simulink model "Simulink_Model"  (R2021a)
settings: Solver=VariableStepAuto  StartTime=0.0  StopTime=inf  FixedStep=1  RelTol=1e-3
model workspace (MAT data in the model file):
  M = 1200
  R = 1
libraries: pid_lib x1, simulink x1
settings Model: EnablePacing=on  Creator=matteopenlington  LastModifiedBy=matteopenlington
settings DebuggingCC: UnderSpecifiedDimensionMsg=warning

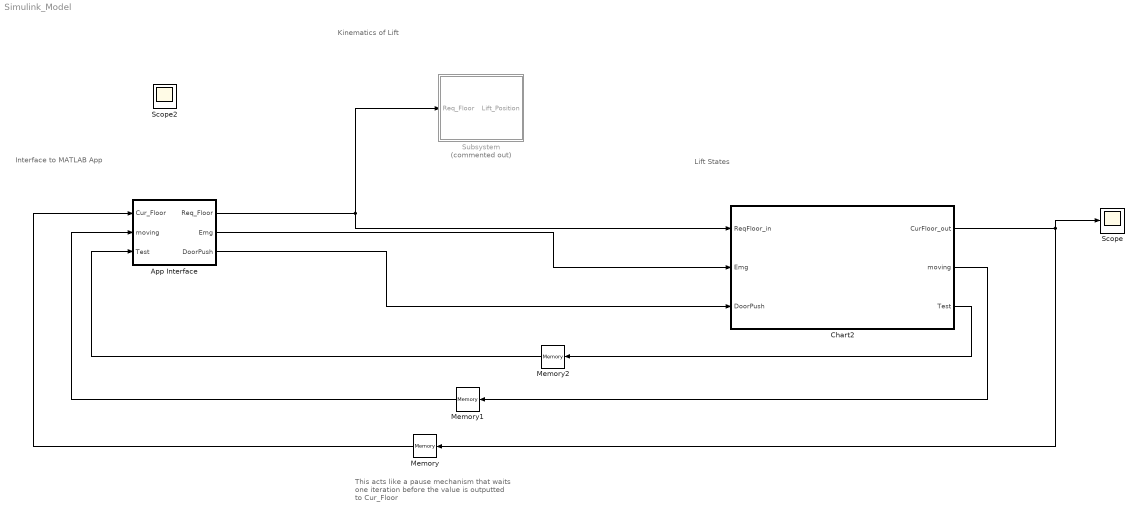
== system Simulink_Model ==
  note: Lift States
  note: Kinematics of Lift
  note: This acts like a pause mechanism that waits one iteration before the value is outputted to Cur_Floor
  note: Interface to MATLAB App
  App Interface : Stateflow chart  TreatAsAtomicUnit=on
  Chart2 : Stateflow chart  TreatAsAtomicUnit=on
  Memory : Memory
  Memory1 : Memory
  Memory2 : Memory
  Scope : Scope
  Subsystem : Subsystem  Commented=on
  Scope2 : Scope
  wires:
  Memory/1 -> App Interface/1(Cur_Floor)
  Chart2/1(CurFloor_out) -> Scope/1, Memory/1
  App Interface/2(Emg) -> Chart2/2(Emg)
  Chart2/2(moving) -> Memory1/1
  Memory1/1 -> App Interface/2(moving)
  App Interface/3(DoorPush) -> Chart2/3(DoorPush)
  Chart2/3(Test) -> Memory2/1
  Memory2/1 -> App Interface/3(Test)
  App Interface/1(Req_Floor) -> Subsystem/1(Req_Floor), Chart2/1(ReqFloor_in)

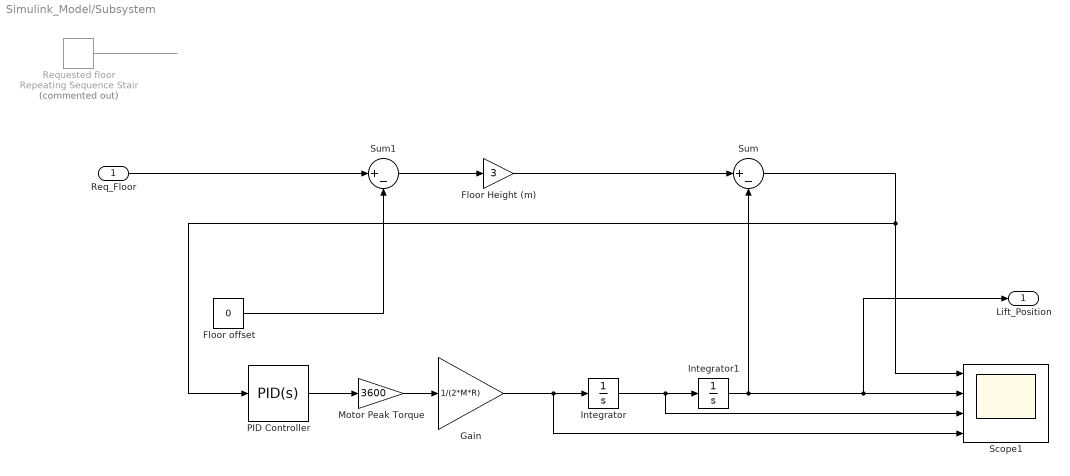
== system Simulink_Model/Subsystem ==
  Req_Floor : Inport
  Floor Height (m) : Gain  Gain=3
  Floor offset : Constant  Value=0
  Gain : Gain  Gain=1/(2*M*R)
  Integrator : Integrator
  Integrator1 : Integrator
  Motor Peak Torque : Gain  Gain=3600
  PID Controller : pid_lib/PID Controller  Controller=PID  Form=Parallel  TimeDomain=Continuous-time  UseExternalTs=off  SampleTime=-1  IntegratorMethod=Forward Euler  FilterMethod=Forward Euler  ControllerParametersSource=internal  P=1  I=0  D=2  UseFilter=on  N=5.45  TunerSelectOption=Transfer Function Based (PID Tuner App)  InitialConditionSource=internal  InitialConditionForIntegrator=0  InitialConditionForFilter=0  DifferentiatorICPrevScaledInput=0  ExternalReset=none  TrackingMode=off  Kt=1  LimitOutput=on  SatLimitsSource=internal  UpperSaturationLimit=1  LowerSaturationLimit=-1  LinearizeAsGain=on  AntiWindupMode=none  Kb=1  POutMin=[]  POutMax=[]  IOutMin=[]  IOutMax=[]  DOutMin=[]  DOutMax=[]  NOutMin=[]  NOutMax=[]  SumOutMin=[]  SumOutMax=[]  SaturationOutMin=[]  SaturationOutMax=[]  PParamMin=[]  PParamMax=[]  IParamMin=[]  IParamMax=[]  DParamMin=[]  DParamMax=[]  NParamMin=[]  NParamMax=[]  KbParamMin=[]  KbParamMax=[]  KtParamMin=[]  KtParamMax=[]  KbOutMin=[]  KbOutMax=[]  KtOutMin=[]  KtOutMax=[]  IntegratorOutMin=[]  IntegratorOutMax=[]  FilterOutMin=[]  FilterOutMax=[]  SumI1OutMin=[]  SumI1OutMax=[]  SumI2OutMin=[]  SumI2OutMax=[]  SumI3OutMin=[]  SumI3OutMax=[]  SumI4OutMin=[]  SumI4OutMax=[]  SumDOutMin=[]  SumDOutMax=[]  DifferentiatorOutMin=[]  DifferentiatorOutMax=[]  FilterDiffOutCoefMin=[]  FilterDiffOutCoefMax=[]  ReciprocalOutMin=[]  ReciprocalOutMax=[]  SumDenOutMin=[]  SumDenOutMax=[]  SumNumOutMin=[]  SumNumOutMax=[]  DivideOutMin=[]  DivideOutMax=[]  UdiffTsProdOutMin=[]  UdiffTsProdOutMax=[]  NTsProdOutMin=[]  NTsProdOutMax=[]  UintegralTsProdOutMin=[]  UintegralTsProdOutMax=[]  UngainTsProdOutMin=[]  UngainTsProdOutMax=[]  IntegratorContinuousStateAttributes=''  IntegratorStateMustResolveToSignalObject=off  IntegratorRTWStateStorageClass=Auto  FilterContinuousStateAttributes=''  FilterStateMustResolveToSignalObject=off  FilterRTWStateStorageClass=Auto  ParallelPVariant=InternalParameters  IdealPVariant=Disabled  IVariant=InternalParameters  DVariant=InternalParameters  IntegratorVariant=Continuous  SatVariant=Enabled  AWVariant=Passthrough  PCopyVariant=Disabled  TRVariant=Disabled  FdbkBlocksVariant=Forward  IdealPFdbkVariant=Disabled  SatFdbkVariant=Disabled  DerivativeFilterVariant=ContFilter  NVariant=InternalParameters  NCopyVariant=Disabled  FilterICVariant=InternalICsFilter  IntegratorICVariant=InternalICs  ExternalResetVariant=Disabled  TRSumVariant=Passthrough  SumFdbkVariant=Disabled  SumVariant=Sum_PID  TsampFilterVariant=InternalTs  TsampNgainVariant=Passthrough  TsampIntegralVariant=Passthrough  ExternalSaturationOutDataTypeStr=Inherit: Same as second input
  Requested floor : simulink/Sources/Repeating Sequence Stair  Commented=on  OutValues=[2:8 5 2 8 7 1].'  tsamp=30  OutMin=[]  OutMax=[]  OutDataTypeStr=double  OutputDataTypeScalingMode=double  OutDataType=fixdt(0,8)  ConRadixGroup=Best Precision: Vector-wise  OutScaling=2^-12
  Scope1 : Scope  NumInputPorts=4
  Sum : Sum  Inputs=|+-
  Sum1 : Sum  Inputs=|+-
  Lift_Position : Outport
  wires:
  Floor offset/1 -> Sum1/2
  Motor Peak Torque/1 -> Gain/1
  Integrator1/1 -> Scope1/2, Lift_Position/1, Sum/2
  Integrator/1 -> Scope1/3, Integrator1/1
  Sum1/1 -> Floor Height (m)/1
  Floor Height (m)/1 -> Sum/1
  PID Controller/1 -> Motor Peak Torque/1
  Sum/1 -> Scope1/1, PID Controller/1
  Gain/1 -> Integrator/1, Scope1/4
  Req_Floor/1 -> Sum1/1
  Requested floor/1 -> ?

== stateflow chart Simulink_Model/App Interface ==
  state InterfaceFromApp
    en:
    coder.extrinsic('AppWSimulink', 'updateCounter', 'Logic', 'Emergency', 'DoorOperation', 'updateDoorStatus');
    app = AppWSimulink(this);
    %Req_Floor = 2;
    initialiseData();
    Logic(app,Req_Floor);
    Emergency(app,Emg);
    DoorOperation(app, DoorPush)
    du:
    if hasChanged(Cur_Floor)
    updateCounter(app, Cur_Floor, Test, Req_Floor);
    end
    if isequal(Cur_Floor, Req_Floor)
    updateDoorStatus(app,Test);
    end
    if (Emg == 1)
    Reset;
    end
    state initialiseData [function]
      (default) -> (junction 12) : {
          | %CurFloor = 0;
          | Req_Floor = 0;
          | Emg = 0;
          | DoorPush =0;
          | }
    state Reset [function]
      (default) -> (junction 119) : {
          | Req_Floor = -10;
          | DoorPush =3;
          | }
  (default) -> InterfaceFromApp
  data: app local; Cur_Floor input; Req_Floor output; Emg output; moving input; DoorPush output; Test input

== stateflow chart Simulink_Model/Chart2 ==
  state No_Error1
    entry:
    CurFloor = 0;
    door = 0;
    hasOpened = 1;
    doorClose = 0;
    Test = -2;
    state Motion [group]
      state MovingUp
        entry:
        moving = 1;
        CurFloor = CurFloor +1;
        exit:
        moving = 0;
      state MovingDown
        entry:
        moving = 1;
        exit:
        CurFloor = CurFloor - 1;
        moving =0;
    state Not_Moving
      entry:
      CurFloor_out = CurFloor;
      NxtFloor;
      state NxtFloor [function]
        (default) -> (junction 99)
        (junction 99) -> (junction 101) [order 1] : [isempty(ReqFloor_in)]{ReqFloor = -10}
        (junction 99) -> (junction 103) [order 2] : {ReqFloor = ReqFloor_in;}
        (junction 101) -> (junction 105)
        (junction 103) -> (junction 105)
      state Idle
        en:
      state Doors
        note: Need to add lift door openclose buttons
        state DoorClosed
          entry:
          Test =3;
          pause(2);
          doorClose = 1;
          exit:
          door = 0;
        state DoorOpening
          en:
          door = 0;
          doorClose = 0;
          Test = 0
          du:
          OpOpening;
        state DoorClosing
          en:
          ObjectDetection;
          Test = 2;
          du:
          ObjectDetection;
          OpClosing;
        state DoorOpen
          entry:
          Test = 1;
          hasOpened = 1;
        note: These door values do not stop at 1.
        DoorOpening -> DoorOpen : [door >= 1]
        DoorClosing -> DoorClosed : [door <= 0]
        DoorOpen -> DoorClosing : after(2,sec)
      (default) -> Idle
      Idle -> DoorOpening [order 1] : [ReqFloor == CurFloor && hasOpened == 0]
    state OpOpening [function]
      (default) -> (junction 217) : [door <= 1]{door = door + 0.1;}
    state ObjectDetection [function]
      (default) -> (junction 195)
      (junction 195) -> (junction 196) [order 1] : [isempty(ReqFloor_in)]{ReqFloor = -10}
      (junction 195) -> (junction 197) [order 2] : {ReqFloor = ReqFloor_in;}
      (junction 196) -> (junction 198)
      (junction 197) -> (junction 198)
    state OpClosing [function]
      (default) -> (junction 231) : {door = door - 0.1;}
    (default) -> Not_Moving
    Not_Moving -> MovingUp [order 1] : [ReqFloor > CurFloor && door == 0]{hasOpened = 0}
    MovingUp -> Not_Moving : after(2,sec)
    Idle -> (junction 180) [order 2]
    (junction 180) -> (junction 177)
    MovingDown -> Not_Moving : after(2,sec)
    (junction 177) -> Not_Moving : after(0.001,sec)
    (junction 182) -> (junction 177)
    Not_Moving -> MovingDown [order 2] : [-2 < ReqFloor && ReqFloor < CurFloor && door == 0]{hasOpened = 0}
    Doors -> (junction 182) : [doorClose == 1]
  state Emergency
    en:
    Test = 0;
    hasOpened = 0;
  (default) -> No_Error1
  No_Error1 -> Emergency : [Emg == 1]
  Emergency -> No_Error1 : [Emg  == 0]
  data: Sensor local =0; CurFloor local; ReqFloor_in input; CurFloor_out output; ReqFloor local; Emg input; moving output; DoorPush input; door local; Test output; hasOpened local; doorClose local
